simulink library "AEMS_Standard_Library"  (R2016b)
settings: Solver=ode45  StartTime=0.0  StopTime=10.0  RelTol=1e-3
undefined symbols (not defined in the file or in its folder): BkPY, carto, Cbx_extegr, Cbx_lpegrsys, Cbx_portegr, Cnx_bnk_nr_conf, Cnx_cyl_nr_conf, ConfigManagement, configuration_management, Cxx_dcm_io_tmr_end_xxxx, Cxx_dcm_rt_tmr_end, Cxx_DID_xxxx_IO_max, Cxx_DID_xxxx_IO_min, Cxx_egrhsofs, Cxx_vmaniegi, DEM_DEBOUNCE_FREEZE, DEM_DTR_CTL_INVISIBLE, DEM_DTR_CTL_NORMAL, Dem_DtrId2_XXX, Dem_DtrId3_XXX, Dem_DtrId4_XXX, Dem_DtrId5_XXX, Dem_DtrId6_XXX, Dem_DtrId7_XXX, Dem_DtrId8_XXX, Dem_DtrId9_XXX, Dem_DtrId_XXX, Dem_EnableConditionId2_XXX, Dem_EnableConditionId3_XXX, Dem_EnableConditionId4_XXX, Dem_EnableConditionId5_XXX, Dem_EnableConditionId6_XXX, Dem_EnableConditionId7_XXX, Dem_EnableConditionId8_XXX, Dem_EnableConditionId_XXX, Dem_EventId, Dem_EventId2_XXX, Dem_EventId3_XXX, Dem_EventId4_XXX, Dem_EventId5_XXX, Dem_EventId6_XXX, Dem_EventId7_XXX, Dem_EventId8_XXX, Dem_EventId9_XXX, Dem_EventId_Device_Faulttype, Dem_EventId_XXX, DEM_IUMPR_GENERAL_DENOMINATOR, DEM_OPCYC_IGNITION, Dem_RatioId2_XXX, Dem_RatioId3_XXX, Dem_RatioId4_XXX, Dem_RatioId5_XXX, Dem_RatioId6_XXX, Dem_RatioId7_XXX, Dem_RatioId8_XXX, Dem_RatioId_XXX, Dem_StorageConditionId2_XXX, Dem_StorageConditionId3_XXX, Dem_StorageConditionId4_XXX, Dem_StorageConditionId5_XXX ... (+65)
libraries: AEMS_Standard_Library x477, simulink x2
(part 29 of 39)

== system AEMS_Standard_Library/SUB/AEMS_DEM_COUNTER_BASED_DEBOUNCE_1D/AEMS_DEM_COUNTER_BASED_DEBOUNCE_CALL ==
  conditionfulfilled : Inport
  prefailed : Inport  Port=2
  prepassed : Inport  Port=3
  reseteventdebounce : Inport  Port=4
  DemDebounceBehavior : Inport  Port=5
  DemCounterFailedThreshold : Inport  Port=6
  DemCounterIncrementStepSize : Inport  Port=7
  DemCounterJumpUp : Inport  Port=8
  DemCounterJumpUpValue : Inport  Port=9
  DemCounterPassedThreshold : Inport  Port=10
  DemCounterDecrementStepSize : Inport  Port=11
  DemCounterJumpDown : Inport  Port=12
  DemCounterJumpDownValue : Inport  Port=13
  Enable : EnablePort
      settings: AttributesFormatString=StatesWhenEnabling = %<StatesWhenEnabling>
  AEMS_DEM_COUNTERBASEDDEBOUNCE : AEMS_Standard_Library/SUB/AEMS_DEM_COUNTERBASEDDEBOUNCE  Tag=[LIB]  eventid=Dem_EventId_Device_Faulttype
      settings: AttributesFormatString=|
      | %<MaskType>
      | EventId: %<eventid>
  debouncevalue : Outport
      settings: AttributesFormatString=<initial=%<InitialOutput>>\n<whendisabled=%<OutputWhenDisabled>>
  failed : Outport  Port=2
      settings: AttributesFormatString=<initial=%<InitialOutput>>\n<whendisabled=%<OutputWhenDisabled>>
  passed : Outport  Port=3
      settings: AttributesFormatString=<initial=%<InitialOutput>>\n<whendisabled=%<OutputWhenDisabled>>
  wires:
  DemCounterJumpDownValue/1 -> AEMS_DEM_COUNTERBASEDDEBOUNCE/13
  DemCounterJumpDown/1 -> AEMS_DEM_COUNTERBASEDDEBOUNCE/12
  DemCounterDecrementStepSize/1 -> AEMS_DEM_COUNTERBASEDDEBOUNCE/11
  DemCounterPassedThreshold/1 -> AEMS_DEM_COUNTERBASEDDEBOUNCE/10
  DemCounterJumpUpValue/1 -> AEMS_DEM_COUNTERBASEDDEBOUNCE/9
  DemCounterJumpUp/1 -> AEMS_DEM_COUNTERBASEDDEBOUNCE/8
  DemCounterIncrementStepSize/1 -> AEMS_DEM_COUNTERBASEDDEBOUNCE/7
  DemCounterFailedThreshold/1 -> AEMS_DEM_COUNTERBASEDDEBOUNCE/6
  DemDebounceBehavior/1 -> AEMS_DEM_COUNTERBASEDDEBOUNCE/5
  reseteventdebounce/1 -> AEMS_DEM_COUNTERBASEDDEBOUNCE/4
  AEMS_DEM_COUNTERBASEDDEBOUNCE/3 -> passed/1
  AEMS_DEM_COUNTERBASEDDEBOUNCE/2 -> failed/1
  AEMS_DEM_COUNTERBASEDDEBOUNCE/1 -> debouncevalue/1
  prefailed/1 -> AEMS_DEM_COUNTERBASEDDEBOUNCE/2
  prepassed/1 -> AEMS_DEM_COUNTERBASEDDEBOUNCE/3
  conditionfulfilled/1 -> AEMS_DEM_COUNTERBASEDDEBOUNCE/1

== system AEMS_Standard_Library/SUB/AEMS_DEM_COUNTER_BASED_DEBOUNCE_2D/AEMS_DEM_COUNTER_BASED_DEBOUNCE_CALL1 ==
  conditionfulfilled : Inport
  prefailed : Inport  Port=2
  prepassed : Inport  Port=3
  reseteventdebounce : Inport  Port=4
  DemDebounceBehavior : Inport  Port=5
  DemCounterFailedThreshold : Inport  Port=6
  DemCounterIncrementStepSize : Inport  Port=7
  DemCounterJumpUp : Inport  Port=8
  DemCounterJumpUpValue : Inport  Port=9
  DemCounterPassedThreshold : Inport  Port=10
  DemCounterDecrementStepSize : Inport  Port=11
  DemCounterJumpDown : Inport  Port=12
  DemCounterJumpDownValue : Inport  Port=13
  Enable : EnablePort
  AEMS_DEM_COUNTERBASEDDEBOUNCE : AEMS_Standard_Library/SUB/AEMS_DEM_COUNTERBASEDDEBOUNCE  Tag=[LIB]  eventid=Dem_EventId_Device_Faulttype
      settings: AttributesFormatString=|
      | %<MaskType>
      | EventId: %<eventid>
  debouncevalue : Outport
  failed : Outport  Port=2
  passed : Outport  Port=3
  wires:
  DemCounterJumpDown/1 -> AEMS_DEM_COUNTERBASEDDEBOUNCE/12
  DemCounterJumpDownValue/1 -> AEMS_DEM_COUNTERBASEDDEBOUNCE/13
  DemDebounceBehavior/1 -> AEMS_DEM_COUNTERBASEDDEBOUNCE/5
  DemCounterFailedThreshold/1 -> AEMS_DEM_COUNTERBASEDDEBOUNCE/6
  DemCounterJumpUpValue/1 -> AEMS_DEM_COUNTERBASEDDEBOUNCE/9
  DemCounterIncrementStepSize/1 -> AEMS_DEM_COUNTERBASEDDEBOUNCE/7
  DemCounterJumpUp/1 -> AEMS_DEM_COUNTERBASEDDEBOUNCE/8
  DemCounterPassedThreshold/1 -> AEMS_DEM_COUNTERBASEDDEBOUNCE/10
  DemCounterDecrementStepSize/1 -> AEMS_DEM_COUNTERBASEDDEBOUNCE/11
  reseteventdebounce/1 -> AEMS_DEM_COUNTERBASEDDEBOUNCE/4
  conditionfulfilled/1 -> AEMS_DEM_COUNTERBASEDDEBOUNCE/1
  prepassed/1 -> AEMS_DEM_COUNTERBASEDDEBOUNCE/3
  prefailed/1 -> AEMS_DEM_COUNTERBASEDDEBOUNCE/2
  AEMS_DEM_COUNTERBASEDDEBOUNCE/1 -> debouncevalue/1
  AEMS_DEM_COUNTERBASEDDEBOUNCE/2 -> failed/1
  AEMS_DEM_COUNTERBASEDDEBOUNCE/3 -> passed/1

== system AEMS_Standard_Library/SUB/AEMS_DEM_COUNTER_BASED_DEBOUNCE_2D/AEMS_DEM_COUNTER_BASED_DEBOUNCE_CALL2 ==
  conditionfulfilled : Inport
  prefailed : Inport  Port=2
  prepassed : Inport  Port=3
  reseteventdebounce : Inport  Port=4
  DemDebounceBehavior : Inport  Port=5
  DemCounterFailedThreshold : Inport  Port=6
  DemCounterIncrementStepSize : Inport  Port=7
  DemCounterJumpUp : Inport  Port=8
  DemCounterJumpUpValue : Inport  Port=9
  DemCounterPassedThreshold : Inport  Port=10
  DemCounterDecrementStepSize : Inport  Port=11
  DemCounterJumpDown : Inport  Port=12
  DemCounterJumpDownValue : Inport  Port=13
  Enable : EnablePort
  AEMS_DEM_COUNTERBASEDDEBOUNCE : AEMS_Standard_Library/SUB/AEMS_DEM_COUNTERBASEDDEBOUNCE  Tag=[LIB]  eventid=Dem_EventId_Device2_Faulttype
      settings: AttributesFormatString=|
      | %<MaskType>
      | EventId: %<eventid>
  debouncevalue : Outport
  failed : Outport  Port=2
  passed : Outport  Port=3
  wires:
  DemCounterJumpDownValue/1 -> AEMS_DEM_COUNTERBASEDDEBOUNCE/13
  DemCounterJumpDown/1 -> AEMS_DEM_COUNTERBASEDDEBOUNCE/12
  DemCounterDecrementStepSize/1 -> AEMS_DEM_COUNTERBASEDDEBOUNCE/11
  DemCounterPassedThreshold/1 -> AEMS_DEM_COUNTERBASEDDEBOUNCE/10
  DemCounterJumpUpValue/1 -> AEMS_DEM_COUNTERBASEDDEBOUNCE/9
  DemCounterJumpUp/1 -> AEMS_DEM_COUNTERBASEDDEBOUNCE/8
  DemCounterIncrementStepSize/1 -> AEMS_DEM_COUNTERBASEDDEBOUNCE/7
  DemCounterFailedThreshold/1 -> AEMS_DEM_COUNTERBASEDDEBOUNCE/6
  DemDebounceBehavior/1 -> AEMS_DEM_COUNTERBASEDDEBOUNCE/5
  reseteventdebounce/1 -> AEMS_DEM_COUNTERBASEDDEBOUNCE/4
  conditionfulfilled/1 -> AEMS_DEM_COUNTERBASEDDEBOUNCE/1
  prepassed/1 -> AEMS_DEM_COUNTERBASEDDEBOUNCE/3
  prefailed/1 -> AEMS_DEM_COUNTERBASEDDEBOUNCE/2
  AEMS_DEM_COUNTERBASEDDEBOUNCE/1 -> debouncevalue/1
  AEMS_DEM_COUNTERBASEDDEBOUNCE/2 -> failed/1
  AEMS_DEM_COUNTERBASEDDEBOUNCE/3 -> passed/1

== system AEMS_Standard_Library/SUB/AEMS_DEM_COUNTER_BASED_DEBOUNCE_3D/AEMS_DEM_COUNTER_BASED_DEBOUNCE_CALL1 ==
  conditionfulfilled : Inport
  prefailed : Inport  Port=2
  prepassed : Inport  Port=3
  reseteventdebounce : Inport  Port=4
  DemDebounceBehavior : Inport  Port=5
  DemCounterFailedThreshold : Inport  Port=6
  DemCounterIncrementStepSize : Inport  Port=7
  DemCounterJumpUp : Inport  Port=8
  DemCounterJumpUpValue : Inport  Port=9
  DemCounterPassedThreshold : Inport  Port=10
  DemCounterDecrementStepSize : Inport  Port=11
  DemCounterJumpDown : Inport  Port=12
  DemCounterJumpDownValue : Inport  Port=13
  Enable : EnablePort
  AEMS_DEM_COUNTERBASEDDEBOUNCE : AEMS_Standard_Library/SUB/AEMS_DEM_COUNTERBASEDDEBOUNCE  Tag=[LIB]  eventid=Dem_EventId_Device_Faulttype
      settings: AttributesFormatString=|
      | %<MaskType>
      | EventId: %<eventid>
  debouncevalue : Outport
  failed : Outport  Port=2
  passed : Outport  Port=3
  wires:
  DemDebounceBehavior/1 -> AEMS_DEM_COUNTERBASEDDEBOUNCE/5
  DemCounterIncrementStepSize/1 -> AEMS_DEM_COUNTERBASEDDEBOUNCE/7
  DemCounterFailedThreshold/1 -> AEMS_DEM_COUNTERBASEDDEBOUNCE/6
  DemCounterJumpUp/1 -> AEMS_DEM_COUNTERBASEDDEBOUNCE/8
  DemCounterPassedThreshold/1 -> AEMS_DEM_COUNTERBASEDDEBOUNCE/10
  DemCounterJumpUpValue/1 -> AEMS_DEM_COUNTERBASEDDEBOUNCE/9
  DemCounterDecrementStepSize/1 -> AEMS_DEM_COUNTERBASEDDEBOUNCE/11
  DemCounterJumpDownValue/1 -> AEMS_DEM_COUNTERBASEDDEBOUNCE/13
  DemCounterJumpDown/1 -> AEMS_DEM_COUNTERBASEDDEBOUNCE/12
  reseteventdebounce/1 -> AEMS_DEM_COUNTERBASEDDEBOUNCE/4
  conditionfulfilled/1 -> AEMS_DEM_COUNTERBASEDDEBOUNCE/1
  prepassed/1 -> AEMS_DEM_COUNTERBASEDDEBOUNCE/3
  prefailed/1 -> AEMS_DEM_COUNTERBASEDDEBOUNCE/2
  AEMS_DEM_COUNTERBASEDDEBOUNCE/1 -> debouncevalue/1
  AEMS_DEM_COUNTERBASEDDEBOUNCE/2 -> failed/1
  AEMS_DEM_COUNTERBASEDDEBOUNCE/3 -> passed/1

== system AEMS_Standard_Library/SUB/AEMS_DEM_COUNTER_BASED_DEBOUNCE_3D/AEMS_DEM_COUNTER_BASED_DEBOUNCE_CALL2 ==
  conditionfulfilled : Inport
  prefailed : Inport  Port=2
  prepassed : Inport  Port=3
  reseteventdebounce : Inport  Port=4
  DemDebounceBehavior : Inport  Port=5
  DemCounterFailedThreshold : Inport  Port=6
  DemCounterIncrementStepSize : Inport  Port=7
  DemCounterJumpUp : Inport  Port=8
  DemCounterJumpUpValue : Inport  Port=9
  DemCounterPassedThreshold : Inport  Port=10
  DemCounterDecrementStepSize : Inport  Port=11
  DemCounterJumpDown : Inport  Port=12
  DemCounterJumpDownValue : Inport  Port=13
  Enable : EnablePort
  AEMS_DEM_COUNTERBASEDDEBOUNCE : AEMS_Standard_Library/SUB/AEMS_DEM_COUNTERBASEDDEBOUNCE  Tag=[LIB]  eventid=Dem_EventId_Device2_Faulttype
      settings: AttributesFormatString=|
      | %<MaskType>
      | EventId: %<eventid>
  debouncevalue : Outport
  failed : Outport  Port=2
  passed : Outport  Port=3
  wires:
  DemDebounceBehavior/1 -> AEMS_DEM_COUNTERBASEDDEBOUNCE/5
  DemCounterIncrementStepSize/1 -> AEMS_DEM_COUNTERBASEDDEBOUNCE/7
  DemCounterFailedThreshold/1 -> AEMS_DEM_COUNTERBASEDDEBOUNCE/6
  DemCounterJumpUp/1 -> AEMS_DEM_COUNTERBASEDDEBOUNCE/8
  DemCounterPassedThreshold/1 -> AEMS_DEM_COUNTERBASEDDEBOUNCE/10
  DemCounterJumpUpValue/1 -> AEMS_DEM_COUNTERBASEDDEBOUNCE/9
  DemCounterDecrementStepSize/1 -> AEMS_DEM_COUNTERBASEDDEBOUNCE/11
  DemCounterJumpDownValue/1 -> AEMS_DEM_COUNTERBASEDDEBOUNCE/13
  DemCounterJumpDown/1 -> AEMS_DEM_COUNTERBASEDDEBOUNCE/12
  reseteventdebounce/1 -> AEMS_DEM_COUNTERBASEDDEBOUNCE/4
  conditionfulfilled/1 -> AEMS_DEM_COUNTERBASEDDEBOUNCE/1
  prepassed/1 -> AEMS_DEM_COUNTERBASEDDEBOUNCE/3
  prefailed/1 -> AEMS_DEM_COUNTERBASEDDEBOUNCE/2
  AEMS_DEM_COUNTERBASEDDEBOUNCE/1 -> debouncevalue/1
  AEMS_DEM_COUNTERBASEDDEBOUNCE/2 -> failed/1
  AEMS_DEM_COUNTERBASEDDEBOUNCE/3 -> passed/1

== system AEMS_Standard_Library/SUB/AEMS_DEM_COUNTER_BASED_DEBOUNCE_3D/AEMS_DEM_COUNTER_BASED_DEBOUNCE_CALL3 ==
  conditionfulfilled : Inport
  prefailed : Inport  Port=2
  prepassed : Inport  Port=3
  reseteventdebounce : Inport  Port=4
  DemDebounceBehavior : Inport  Port=5
  DemCounterFailedThreshold : Inport  Port=6
  DemCounterIncrementStepSize : Inport  Port=7
  DemCounterJumpUp : Inport  Port=8
  DemCounterJumpUpValue : Inport  Port=9
  DemCounterPassedThreshold : Inport  Port=10
  DemCounterDecrementStepSize : Inport  Port=11
  DemCounterJumpDown : Inport  Port=12
  DemCounterJumpDownValue : Inport  Port=13
  Enable : EnablePort
  AEMS_DEM_COUNTERBASEDDEBOUNCE : AEMS_Standard_Library/SUB/AEMS_DEM_COUNTERBASEDDEBOUNCE  Tag=[LIB]  eventid=Dem_EventId_Device3_Faulttype
      settings: AttributesFormatString=|
      | %<MaskType>
      | EventId: %<eventid>
  debouncevalue : Outport
  failed : Outport  Port=2
  passed : Outport  Port=3
  wires:
  DemCounterJumpDownValue/1 -> AEMS_DEM_COUNTERBASEDDEBOUNCE/13
  DemDebounceBehavior/1 -> AEMS_DEM_COUNTERBASEDDEBOUNCE/5
  DemCounterFailedThreshold/1 -> AEMS_DEM_COUNTERBASEDDEBOUNCE/6
  DemCounterIncrementStepSize/1 -> AEMS_DEM_COUNTERBASEDDEBOUNCE/7
  DemCounterJumpUp/1 -> AEMS_DEM_COUNTERBASEDDEBOUNCE/8
  DemCounterJumpUpValue/1 -> AEMS_DEM_COUNTERBASEDDEBOUNCE/9
  DemCounterPassedThreshold/1 -> AEMS_DEM_COUNTERBASEDDEBOUNCE/10
  DemCounterDecrementStepSize/1 -> AEMS_DEM_COUNTERBASEDDEBOUNCE/11
  DemCounterJumpDown/1 -> AEMS_DEM_COUNTERBASEDDEBOUNCE/12
  reseteventdebounce/1 -> AEMS_DEM_COUNTERBASEDDEBOUNCE/4
  AEMS_DEM_COUNTERBASEDDEBOUNCE/3 -> passed/1
  AEMS_DEM_COUNTERBASEDDEBOUNCE/2 -> failed/1
  AEMS_DEM_COUNTERBASEDDEBOUNCE/1 -> debouncevalue/1
  prefailed/1 -> AEMS_DEM_COUNTERBASEDDEBOUNCE/2
  prepassed/1 -> AEMS_DEM_COUNTERBASEDDEBOUNCE/3
  conditionfulfilled/1 -> AEMS_DEM_COUNTERBASEDDEBOUNCE/1

== system AEMS_Standard_Library/SUB/AEMS_DEM_COUNTER_BASED_DEBOUNCE_4D/AEMS_DEM_COUNTER_BASED_DEBOUNCE_CALL1 ==
  conditionfulfilled : Inport
  prefailed : Inport  Port=2
  prepassed : Inport  Port=3
  reseteventdebounce : Inport  Port=4
  DemDebounceBehavior : Inport  Port=5
  DemCounterFailedThreshold : Inport  Port=6
  DemCounterIncrementStepSize : Inport  Port=7
  DemCounterJumpUp : Inport  Port=8
  DemCounterJumpUpValue : Inport  Port=9
  DemCounterPassedThreshold : Inport  Port=10
  DemCounterDecrementStepSize : Inport  Port=11
  DemCounterJumpDown : Inport  Port=12
  DemCounterJumpDownValue : Inport  Port=13
  Enable : EnablePort
  AEMS_DEM_COUNTERBASEDDEBOUNCE : AEMS_Standard_Library/SUB/AEMS_DEM_COUNTERBASEDDEBOUNCE  Tag=[LIB]  eventid=Dem_EventId_Device_Faulttype
      settings: AttributesFormatString=|
      | %<MaskType>
      | EventId: %<eventid>
  debouncevalue : Outport
  failed : Outport  Port=2
  passed : Outport  Port=3
  wires:
  reseteventdebounce/1 -> AEMS_DEM_COUNTERBASEDDEBOUNCE/4
  DemCounterIncrementStepSize/1 -> AEMS_DEM_COUNTERBASEDDEBOUNCE/7
  DemCounterJumpUpValue/1 -> AEMS_DEM_COUNTERBASEDDEBOUNCE/9
  DemDebounceBehavior/1 -> AEMS_DEM_COUNTERBASEDDEBOUNCE/5
  DemCounterJumpUp/1 -> AEMS_DEM_COUNTERBASEDDEBOUNCE/8
  DemCounterDecrementStepSize/1 -> AEMS_DEM_COUNTERBASEDDEBOUNCE/11
  DemCounterPassedThreshold/1 -> AEMS_DEM_COUNTERBASEDDEBOUNCE/10
  DemCounterFailedThreshold/1 -> AEMS_DEM_COUNTERBASEDDEBOUNCE/6
  DemCounterJumpDown/1 -> AEMS_DEM_COUNTERBASEDDEBOUNCE/12
  DemCounterJumpDownValue/1 -> AEMS_DEM_COUNTERBASEDDEBOUNCE/13
  AEMS_DEM_COUNTERBASEDDEBOUNCE/3 -> passed/1
  AEMS_DEM_COUNTERBASEDDEBOUNCE/2 -> failed/1
  AEMS_DEM_COUNTERBASEDDEBOUNCE/1 -> debouncevalue/1
  prefailed/1 -> AEMS_DEM_COUNTERBASEDDEBOUNCE/2
  prepassed/1 -> AEMS_DEM_COUNTERBASEDDEBOUNCE/3
  conditionfulfilled/1 -> AEMS_DEM_COUNTERBASEDDEBOUNCE/1

== system AEMS_Standard_Library/SUB/AEMS_DEM_COUNTER_BASED_DEBOUNCE_4D/AEMS_DEM_COUNTER_BASED_DEBOUNCE_CALL2 ==
  conditionfulfilled : Inport
  prefailed : Inport  Port=2
  prepassed : Inport  Port=3
  reseteventdebounce : Inport  Port=4
  DemDebounceBehavior : Inport  Port=5
  DemCounterFailedThreshold : Inport  Port=6
  DemCounterIncrementStepSize : Inport  Port=7
  DemCounterJumpUp : Inport  Port=8
  DemCounterJumpUpValue : Inport  Port=9
  DemCounterPassedThreshold : Inport  Port=10
  DemCounterDecrementStepSize : Inport  Port=11
  DemCounterJumpDown : Inport  Port=12
  DemCounterJumpDownValue : Inport  Port=13
  Enable : EnablePort
  AEMS_DEM_COUNTERBASEDDEBOUNCE : AEMS_Standard_Library/SUB/AEMS_DEM_COUNTERBASEDDEBOUNCE  Tag=[LIB]  eventid=Dem_EventId_Device2_Faulttype
      settings: AttributesFormatString=|
      | %<MaskType>
      | EventId: %<eventid>
  debouncevalue : Outport
  failed : Outport  Port=2
  passed : Outport  Port=3
  wires:
  DemCounterIncrementStepSize/1 -> AEMS_DEM_COUNTERBASEDDEBOUNCE/7
  DemDebounceBehavior/1 -> AEMS_DEM_COUNTERBASEDDEBOUNCE/5
  DemCounterJumpUpValue/1 -> AEMS_DEM_COUNTERBASEDDEBOUNCE/9
  DemCounterFailedThreshold/1 -> AEMS_DEM_COUNTERBASEDDEBOUNCE/6
  DemCounterJumpUp/1 -> AEMS_DEM_COUNTERBASEDDEBOUNCE/8
  DemCounterDecrementStepSize/1 -> AEMS_DEM_COUNTERBASEDDEBOUNCE/11
  DemCounterPassedThreshold/1 -> AEMS_DEM_COUNTERBASEDDEBOUNCE/10
  DemCounterJumpDownValue/1 -> AEMS_DEM_COUNTERBASEDDEBOUNCE/13
  DemCounterJumpDown/1 -> AEMS_DEM_COUNTERBASEDDEBOUNCE/12
  reseteventdebounce/1 -> AEMS_DEM_COUNTERBASEDDEBOUNCE/4
  AEMS_DEM_COUNTERBASEDDEBOUNCE/3 -> passed/1
  AEMS_DEM_COUNTERBASEDDEBOUNCE/2 -> failed/1
  AEMS_DEM_COUNTERBASEDDEBOUNCE/1 -> debouncevalue/1
  prefailed/1 -> AEMS_DEM_COUNTERBASEDDEBOUNCE/2
  prepassed/1 -> AEMS_DEM_COUNTERBASEDDEBOUNCE/3
  conditionfulfilled/1 -> AEMS_DEM_COUNTERBASEDDEBOUNCE/1

== system AEMS_Standard_Library/SUB/AEMS_DEM_COUNTER_BASED_DEBOUNCE_4D/AEMS_DEM_COUNTER_BASED_DEBOUNCE_CALL3 ==
  conditionfulfilled : Inport
  prefailed : Inport  Port=2
  prepassed : Inport  Port=3
  reseteventdebounce : Inport  Port=4
  DemDebounceBehavior : Inport  Port=5
  DemCounterFailedThreshold : Inport  Port=6
  DemCounterIncrementStepSize : Inport  Port=7
  DemCounterJumpUp : Inport  Port=8
  DemCounterJumpUpValue : Inport  Port=9
  DemCounterPassedThreshold : Inport  Port=10
  DemCounterDecrementStepSize : Inport  Port=11
  DemCounterJumpDown : Inport  Port=12
  DemCounterJumpDownValue : Inport  Port=13
  Enable : EnablePort
  AEMS_DEM_COUNTERBASEDDEBOUNCE : AEMS_Standard_Library/SUB/AEMS_DEM_COUNTERBASEDDEBOUNCE  Tag=[LIB]  eventid=Dem_EventId_Device3_Faulttype
      settings: AttributesFormatString=|
      | %<MaskType>
      | EventId: %<eventid>
  debouncevalue : Outport
  failed : Outport  Port=2
  passed : Outport  Port=3
  wires:
  reseteventdebounce/1 -> AEMS_DEM_COUNTERBASEDDEBOUNCE/4
  DemCounterJumpDown/1 -> AEMS_DEM_COUNTERBASEDDEBOUNCE/12
  DemCounterPassedThreshold/1 -> AEMS_DEM_COUNTERBASEDDEBOUNCE/10
  DemDebounceBehavior/1 -> AEMS_DEM_COUNTERBASEDDEBOUNCE/5
  DemCounterJumpUpValue/1 -> AEMS_DEM_COUNTERBASEDDEBOUNCE/9
  DemCounterDecrementStepSize/1 -> AEMS_DEM_COUNTERBASEDDEBOUNCE/11
  DemCounterFailedThreshold/1 -> AEMS_DEM_COUNTERBASEDDEBOUNCE/6
  DemCounterIncrementStepSize/1 -> AEMS_DEM_COUNTERBASEDDEBOUNCE/7
  DemCounterJumpDownValue/1 -> AEMS_DEM_COUNTERBASEDDEBOUNCE/13
  DemCounterJumpUp/1 -> AEMS_DEM_COUNTERBASEDDEBOUNCE/8
  conditionfulfilled/1 -> AEMS_DEM_COUNTERBASEDDEBOUNCE/1
  prepassed/1 -> AEMS_DEM_COUNTERBASEDDEBOUNCE/3
  prefailed/1 -> AEMS_DEM_COUNTERBASEDDEBOUNCE/2
  AEMS_DEM_COUNTERBASEDDEBOUNCE/1 -> debouncevalue/1
  AEMS_DEM_COUNTERBASEDDEBOUNCE/2 -> failed/1
  AEMS_DEM_COUNTERBASEDDEBOUNCE/3 -> passed/1

== system AEMS_Standard_Library/SUB/AEMS_DEM_COUNTER_BASED_DEBOUNCE_4D/AEMS_DEM_COUNTER_BASED_DEBOUNCE_CALL4 ==
  conditionfulfilled : Inport
  prefailed : Inport  Port=2
  prepassed : Inport  Port=3
  reseteventdebounce : Inport  Port=4
  DemDebounceBehavior : Inport  Port=5
  DemCounterFailedThreshold : Inport  Port=6
  DemCounterIncrementStepSize : Inport  Port=7
  DemCounterJumpUp : Inport  Port=8
  DemCounterJumpUpValue : Inport  Port=9
  DemCounterPassedThreshold : Inport  Port=10
  DemCounterDecrementStepSize : Inport  Port=11
  DemCounterJumpDown : Inport  Port=12
  DemCounterJumpDownValue : Inport  Port=13
  Enable : EnablePort
  AEMS_DEM_COUNTERBASEDDEBOUNCE : AEMS_Standard_Library/SUB/AEMS_DEM_COUNTERBASEDDEBOUNCE  Tag=[LIB]  eventid=Dem_EventId_Device4_Faulttype
      settings: AttributesFormatString=|
      | %<MaskType>
      | EventId: %<eventid>
  debouncevalue : Outport
  failed : Outport  Port=2
  passed : Outport  Port=3
  wires:
  DemCounterDecrementStepSize/1 -> AEMS_DEM_COUNTERBASEDDEBOUNCE/11
  DemCounterJumpDown/1 -> AEMS_DEM_COUNTERBASEDDEBOUNCE/12
  DemDebounceBehavior/1 -> AEMS_DEM_COUNTERBASEDDEBOUNCE/5
  DemCounterFailedThreshold/1 -> AEMS_DEM_COUNTERBASEDDEBOUNCE/6
  reseteventdebounce/1 -> AEMS_DEM_COUNTERBASEDDEBOUNCE/4
  DemCounterIncrementStepSize/1 -> AEMS_DEM_COUNTERBASEDDEBOUNCE/7
  DemCounterJumpUpValue/1 -> AEMS_DEM_COUNTERBASEDDEBOUNCE/9
  DemCounterJumpDownValue/1 -> AEMS_DEM_COUNTERBASEDDEBOUNCE/13
  DemCounterJumpUp/1 -> AEMS_DEM_COUNTERBASEDDEBOUNCE/8
  DemCounterPassedThreshold/1 -> AEMS_DEM_COUNTERBASEDDEBOUNCE/10
  AEMS_DEM_COUNTERBASEDDEBOUNCE/3 -> passed/1
  AEMS_DEM_COUNTERBASEDDEBOUNCE/2 -> failed/1
  AEMS_DEM_COUNTERBASEDDEBOUNCE/1 -> debouncevalue/1
  prefailed/1 -> AEMS_DEM_COUNTERBASEDDEBOUNCE/2
  prepassed/1 -> AEMS_DEM_COUNTERBASEDDEBOUNCE/3
  conditionfulfilled/1 -> AEMS_DEM_COUNTERBASEDDEBOUNCE/1

== system AEMS_Standard_Library/SUB/AEMS_DEM_COUNTER_BASED_DEBOUNCE_6D/AEMS_DEM_COUNTER_BASED_DEBOUNCE_CALL1 ==
  conditionfulfilled : Inport
  prefailed : Inport  Port=2
  prepassed : Inport  Port=3
  reseteventdebounce : Inport  Port=4
  DemDebounceBehavior : Inport  Port=5
  DemCounterFailedThreshold : Inport  Port=6
  DemCounterIncrementStepSize : Inport  Port=7
  DemCounterJumpUp : Inport  Port=8
  DemCounterJumpUpValue : Inport  Port=9
  DemCounterPassedThreshold : Inport  Port=10
  DemCounterDecrementStepSize : Inport  Port=11
  DemCounterJumpDown : Inport  Port=12
  DemCounterJumpDownValue : Inport  Port=13
  Enable : EnablePort
  AEMS_DEM_COUNTERBASEDDEBOUNCE : AEMS_Standard_Library/SUB/AEMS_DEM_COUNTERBASEDDEBOUNCE  Tag=[LIB]  eventid=Dem_EventId_Device_Faulttype
      settings: AttributesFormatString=|
      | %<MaskType>
      | EventId: %<eventid>
  debouncevalue : Outport
  failed : Outport  Port=2
  passed : Outport  Port=3
  wires:
  DemCounterJumpUp/1 -> AEMS_DEM_COUNTERBASEDDEBOUNCE/8
  DemCounterIncrementStepSize/1 -> AEMS_DEM_COUNTERBASEDDEBOUNCE/7
  DemCounterJumpUpValue/1 -> AEMS_DEM_COUNTERBASEDDEBOUNCE/9
  DemCounterFailedThreshold/1 -> AEMS_DEM_COUNTERBASEDDEBOUNCE/6
  DemDebounceBehavior/1 -> AEMS_DEM_COUNTERBASEDDEBOUNCE/5
  DemCounterJumpDownValue/1 -> AEMS_DEM_COUNTERBASEDDEBOUNCE/13
  DemCounterJumpDown/1 -> AEMS_DEM_COUNTERBASEDDEBOUNCE/12
  DemCounterDecrementStepSize/1 -> AEMS_DEM_COUNTERBASEDDEBOUNCE/11
  DemCounterPassedThreshold/1 -> AEMS_DEM_COUNTERBASEDDEBOUNCE/10
  reseteventdebounce/1 -> AEMS_DEM_COUNTERBASEDDEBOUNCE/4
  AEMS_DEM_COUNTERBASEDDEBOUNCE/3 -> passed/1
  AEMS_DEM_COUNTERBASEDDEBOUNCE/2 -> failed/1
  AEMS_DEM_COUNTERBASEDDEBOUNCE/1 -> debouncevalue/1
  prefailed/1 -> AEMS_DEM_COUNTERBASEDDEBOUNCE/2
  prepassed/1 -> AEMS_DEM_COUNTERBASEDDEBOUNCE/3
  conditionfulfilled/1 -> AEMS_DEM_COUNTERBASEDDEBOUNCE/1

== system AEMS_Standard_Library/SUB/AEMS_DEM_COUNTER_BASED_DEBOUNCE_6D/AEMS_DEM_COUNTER_BASED_DEBOUNCE_CALL2 ==
  conditionfulfilled : Inport
  prefailed : Inport  Port=2
  prepassed : Inport  Port=3
  reseteventdebounce : Inport  Port=4
  DemDebounceBehavior : Inport  Port=5
  DemCounterFailedThreshold : Inport  Port=6
  DemCounterIncrementStepSize : Inport  Port=7
  DemCounterJumpUp : Inport  Port=8
  DemCounterJumpUpValue : Inport  Port=9
  DemCounterPassedThreshold : Inport  Port=10
  DemCounterDecrementStepSize : Inport  Port=11
  DemCounterJumpDown : Inport  Port=12
  DemCounterJumpDownValue : Inport  Port=13
  Enable : EnablePort
  AEMS_DEM_COUNTERBASEDDEBOUNCE : AEMS_Standard_Library/SUB/AEMS_DEM_COUNTERBASEDDEBOUNCE  Tag=[LIB]  eventid=Dem_EventId_Device2_Faulttype
      settings: AttributesFormatString=|
      | %<MaskType>
      | EventId: %<eventid>
  debouncevalue : Outport
  failed : Outport  Port=2
  passed : Outport  Port=3
  wires:
  reseteventdebounce/1 -> AEMS_DEM_COUNTERBASEDDEBOUNCE/4
  DemCounterJumpDownValue/1 -> AEMS_DEM_COUNTERBASEDDEBOUNCE/13
  DemCounterJumpDown/1 -> AEMS_DEM_COUNTERBASEDDEBOUNCE/12
  DemCounterDecrementStepSize/1 -> AEMS_DEM_COUNTERBASEDDEBOUNCE/11
  DemCounterPassedThreshold/1 -> AEMS_DEM_COUNTERBASEDDEBOUNCE/10
  DemCounterJumpUpValue/1 -> AEMS_DEM_COUNTERBASEDDEBOUNCE/9
  DemCounterJumpUp/1 -> AEMS_DEM_COUNTERBASEDDEBOUNCE/8
  DemCounterIncrementStepSize/1 -> AEMS_DEM_COUNTERBASEDDEBOUNCE/7
  DemCounterFailedThreshold/1 -> AEMS_DEM_COUNTERBASEDDEBOUNCE/6
  DemDebounceBehavior/1 -> AEMS_DEM_COUNTERBASEDDEBOUNCE/5
  AEMS_DEM_COUNTERBASEDDEBOUNCE/3 -> passed/1
  AEMS_DEM_COUNTERBASEDDEBOUNCE/2 -> failed/1
  AEMS_DEM_COUNTERBASEDDEBOUNCE/1 -> debouncevalue/1
  prefailed/1 -> AEMS_DEM_COUNTERBASEDDEBOUNCE/2
  prepassed/1 -> AEMS_DEM_COUNTERBASEDDEBOUNCE/3
  conditionfulfilled/1 -> AEMS_DEM_COUNTERBASEDDEBOUNCE/1

== system AEMS_Standard_Library/SUB/AEMS_DEM_COUNTER_BASED_DEBOUNCE_6D/AEMS_DEM_COUNTER_BASED_DEBOUNCE_CALL3 ==
  conditionfulfilled : Inport
  prefailed : Inport  Port=2
  prepassed : Inport  Port=3
  reseteventdebounce : Inport  Port=4
  DemDebounceBehavior : Inport  Port=5
  DemCounterFailedThreshold : Inport  Port=6
  DemCounterIncrementStepSize : Inport  Port=7
  DemCounterJumpUp : Inport  Port=8
  DemCounterJumpUpValue : Inport  Port=9
  DemCounterPassedThreshold : Inport  Port=10
  DemCounterDecrementStepSize : Inport  Port=11
  DemCounterJumpDown : Inport  Port=12
  DemCounterJumpDownValue : Inport  Port=13
  Enable : EnablePort
  AEMS_DEM_COUNTERBASEDDEBOUNCE : AEMS_Standard_Library/SUB/AEMS_DEM_COUNTERBASEDDEBOUNCE  Tag=[LIB]  eventid=Dem_EventId_Device3_Faulttype
      settings: AttributesFormatString=|
      | %<MaskType>
      | EventId: %<eventid>
  debouncevalue : Outport
  failed : Outport  Port=2
  passed : Outport  Port=3
  wires:
  DemCounterJumpDownValue/1 -> AEMS_DEM_COUNTERBASEDDEBOUNCE/13
  DemCounterJumpDown/1 -> AEMS_DEM_COUNTERBASEDDEBOUNCE/12
  DemCounterDecrementStepSize/1 -> AEMS_DEM_COUNTERBASEDDEBOUNCE/11
  DemCounterPassedThreshold/1 -> AEMS_DEM_COUNTERBASEDDEBOUNCE/10
  DemCounterJumpUpValue/1 -> AEMS_DEM_COUNTERBASEDDEBOUNCE/9
  DemCounterJumpUp/1 -> AEMS_DEM_COUNTERBASEDDEBOUNCE/8
  DemCounterIncrementStepSize/1 -> AEMS_DEM_COUNTERBASEDDEBOUNCE/7
  DemCounterFailedThreshold/1 -> AEMS_DEM_COUNTERBASEDDEBOUNCE/6
  DemDebounceBehavior/1 -> AEMS_DEM_COUNTERBASEDDEBOUNCE/5
  reseteventdebounce/1 -> AEMS_DEM_COUNTERBASEDDEBOUNCE/4
  conditionfulfilled/1 -> AEMS_DEM_COUNTERBASEDDEBOUNCE/1
  prepassed/1 -> AEMS_DEM_COUNTERBASEDDEBOUNCE/3
  prefailed/1 -> AEMS_DEM_COUNTERBASEDDEBOUNCE/2
  AEMS_DEM_COUNTERBASEDDEBOUNCE/1 -> debouncevalue/1
  AEMS_DEM_COUNTERBASEDDEBOUNCE/2 -> failed/1
  AEMS_DEM_COUNTERBASEDDEBOUNCE/3 -> passed/1

== system AEMS_Standard_Library/SUB/AEMS_DEM_COUNTER_BASED_DEBOUNCE_6D/AEMS_DEM_COUNTER_BASED_DEBOUNCE_CALL4 ==
  conditionfulfilled : Inport
  prefailed : Inport  Port=2
  prepassed : Inport  Port=3
  reseteventdebounce : Inport  Port=4
  DemDebounceBehavior : Inport  Port=5
  DemCounterFailedThreshold : Inport  Port=6
  DemCounterIncrementStepSize : Inport  Port=7
  DemCounterJumpUp : Inport  Port=8
  DemCounterJumpUpValue : Inport  Port=9
  DemCounterPassedThreshold : Inport  Port=10
  DemCounterDecrementStepSize : Inport  Port=11
  DemCounterJumpDown : Inport  Port=12
  DemCounterJumpDownValue : Inport  Port=13
  Enable : EnablePort
  AEMS_DEM_COUNTERBASEDDEBOUNCE : AEMS_Standard_Library/SUB/AEMS_DEM_COUNTERBASEDDEBOUNCE  Tag=[LIB]  eventid=Dem_EventId_Device4_Faulttype
      settings: AttributesFormatString=|
      | %<MaskType>
      | EventId: %<eventid>
  debouncevalue : Outport
  failed : Outport  Port=2
  passed : Outport  Port=3
  wires:
  DemCounterJumpDownValue/1 -> AEMS_DEM_COUNTERBASEDDEBOUNCE/13
  DemCounterJumpDown/1 -> AEMS_DEM_COUNTERBASEDDEBOUNCE/12
  DemCounterDecrementStepSize/1 -> AEMS_DEM_COUNTERBASEDDEBOUNCE/11
  DemCounterPassedThreshold/1 -> AEMS_DEM_COUNTERBASEDDEBOUNCE/10
  DemCounterJumpUpValue/1 -> AEMS_DEM_COUNTERBASEDDEBOUNCE/9
  DemCounterJumpUp/1 -> AEMS_DEM_COUNTERBASEDDEBOUNCE/8
  DemCounterIncrementStepSize/1 -> AEMS_DEM_COUNTERBASEDDEBOUNCE/7
  DemCounterFailedThreshold/1 -> AEMS_DEM_COUNTERBASEDDEBOUNCE/6
  DemDebounceBehavior/1 -> AEMS_DEM_COUNTERBASEDDEBOUNCE/5
  reseteventdebounce/1 -> AEMS_DEM_COUNTERBASEDDEBOUNCE/4
  AEMS_DEM_COUNTERBASEDDEBOUNCE/3 -> passed/1
  AEMS_DEM_COUNTERBASEDDEBOUNCE/2 -> failed/1
  AEMS_DEM_COUNTERBASEDDEBOUNCE/1 -> debouncevalue/1
  prefailed/1 -> AEMS_DEM_COUNTERBASEDDEBOUNCE/2
  prepassed/1 -> AEMS_DEM_COUNTERBASEDDEBOUNCE/3
  conditionfulfilled/1 -> AEMS_DEM_COUNTERBASEDDEBOUNCE/1

== system AEMS_Standard_Library/SUB/AEMS_DEM_COUNTER_BASED_DEBOUNCE_6D/AEMS_DEM_COUNTER_BASED_DEBOUNCE_CALL5 ==
  conditionfulfilled : Inport
  prefailed : Inport  Port=2
  prepassed : Inport  Port=3
  reseteventdebounce : Inport  Port=4
  DemDebounceBehavior : Inport  Port=5
  DemCounterFailedThreshold : Inport  Port=6
  DemCounterIncrementStepSize : Inport  Port=7
  DemCounterJumpUp : Inport  Port=8
  DemCounterJumpUpValue : Inport  Port=9
  DemCounterPassedThreshold : Inport  Port=10
  DemCounterDecrementStepSize : Inport  Port=11
  DemCounterJumpDown : Inport  Port=12
  DemCounterJumpDownValue : Inport  Port=13
  Enable : EnablePort
  AEMS_DEM_COUNTERBASEDDEBOUNCE : AEMS_Standard_Library/SUB/AEMS_DEM_COUNTERBASEDDEBOUNCE  Tag=[LIB]  eventid=Dem_EventId_Device5_Faulttype
      settings: AttributesFormatString=|
      | %<MaskType>
      | EventId: %<eventid>
  debouncevalue : Outport
  failed : Outport  Port=2
  passed : Outport  Port=3
  wires:
  DemCounterJumpDownValue/1 -> AEMS_DEM_COUNTERBASEDDEBOUNCE/13
  DemCounterJumpDown/1 -> AEMS_DEM_COUNTERBASEDDEBOUNCE/12
  DemCounterDecrementStepSize/1 -> AEMS_DEM_COUNTERBASEDDEBOUNCE/11
  DemCounterPassedThreshold/1 -> AEMS_DEM_COUNTERBASEDDEBOUNCE/10
  DemCounterJumpUpValue/1 -> AEMS_DEM_COUNTERBASEDDEBOUNCE/9
  DemCounterJumpUp/1 -> AEMS_DEM_COUNTERBASEDDEBOUNCE/8
  DemCounterIncrementStepSize/1 -> AEMS_DEM_COUNTERBASEDDEBOUNCE/7
  DemCounterFailedThreshold/1 -> AEMS_DEM_COUNTERBASEDDEBOUNCE/6
  DemDebounceBehavior/1 -> AEMS_DEM_COUNTERBASEDDEBOUNCE/5
  reseteventdebounce/1 -> AEMS_DEM_COUNTERBASEDDEBOUNCE/4
  AEMS_DEM_COUNTERBASEDDEBOUNCE/3 -> passed/1
  AEMS_DEM_COUNTERBASEDDEBOUNCE/2 -> failed/1
  AEMS_DEM_COUNTERBASEDDEBOUNCE/1 -> debouncevalue/1
  prefailed/1 -> AEMS_DEM_COUNTERBASEDDEBOUNCE/2
  prepassed/1 -> AEMS_DEM_COUNTERBASEDDEBOUNCE/3
  conditionfulfilled/1 -> AEMS_DEM_COUNTERBASEDDEBOUNCE/1

== system AEMS_Standard_Library/SUB/AEMS_DEM_COUNTER_BASED_DEBOUNCE_6D/AEMS_DEM_COUNTER_BASED_DEBOUNCE_CALL6 ==
  conditionfulfilled : Inport
  prefailed : Inport  Port=2
  prepassed : Inport  Port=3
  reseteventdebounce : Inport  Port=4
  DemDebounceBehavior : Inport  Port=5
  DemCounterFailedThreshold : Inport  Port=6
  DemCounterIncrementStepSize : Inport  Port=7
  DemCounterJumpUp : Inport  Port=8
  DemCounterJumpUpValue : Inport  Port=9
  DemCounterPassedThreshold : Inport  Port=10
  DemCounterDecrementStepSize : Inport  Port=11
  DemCounterJumpDown : Inport  Port=12
  DemCounterJumpDownValue : Inport  Port=13
  Enable : EnablePort
  AEMS_DEM_COUNTERBASEDDEBOUNCE : AEMS_Standard_Library/SUB/AEMS_DEM_COUNTERBASEDDEBOUNCE  Tag=[LIB]  eventid=Dem_EventId_Device6_Faulttype
      settings: AttributesFormatString=|
      | %<MaskType>
      | EventId: %<eventid>
  debouncevalue : Outport
  failed : Outport  Port=2
  passed : Outport  Port=3
  wires:
  DemCounterJumpDownValue/1 -> AEMS_DEM_COUNTERBASEDDEBOUNCE/13
  DemCounterJumpDown/1 -> AEMS_DEM_COUNTERBASEDDEBOUNCE/12
  DemCounterDecrementStepSize/1 -> AEMS_DEM_COUNTERBASEDDEBOUNCE/11
  DemCounterPassedThreshold/1 -> AEMS_DEM_COUNTERBASEDDEBOUNCE/10
  DemCounterJumpUpValue/1 -> AEMS_DEM_COUNTERBASEDDEBOUNCE/9
  DemCounterJumpUp/1 -> AEMS_DEM_COUNTERBASEDDEBOUNCE/8
  DemCounterIncrementStepSize/1 -> AEMS_DEM_COUNTERBASEDDEBOUNCE/7
  DemCounterFailedThreshold/1 -> AEMS_DEM_COUNTERBASEDDEBOUNCE/6
  DemDebounceBehavior/1 -> AEMS_DEM_COUNTERBASEDDEBOUNCE/5
  reseteventdebounce/1 -> AEMS_DEM_COUNTERBASEDDEBOUNCE/4
  AEMS_DEM_COUNTERBASEDDEBOUNCE/3 -> passed/1
  AEMS_DEM_COUNTERBASEDDEBOUNCE/2 -> failed/1
  AEMS_DEM_COUNTERBASEDDEBOUNCE/1 -> debouncevalue/1
  prefailed/1 -> AEMS_DEM_COUNTERBASEDDEBOUNCE/2
  prepassed/1 -> AEMS_DEM_COUNTERBASEDDEBOUNCE/3
  conditionfulfilled/1 -> AEMS_DEM_COUNTERBASEDDEBOUNCE/1

== system AEMS_Standard_Library/SUB/AEMS_DEM_COUNTER_BASED_DEBOUNCE_8D/AEMS_DEM_COUNTER_BASED_DEBOUNCE_CALL1 ==
  conditionfulfilled : Inport
  prefailed : Inport  Port=2
  prepassed : Inport  Port=3
  reseteventdebounce : Inport  Port=4
  DemDebounceBehavior : Inport  Port=5
  DemCounterFailedThreshold : Inport  Port=6
  DemCounterIncrementStepSize : Inport  Port=7
  DemCounterJumpUp : Inport  Port=8
  DemCounterJumpUpValue : Inport  Port=9
  DemCounterPassedThreshold : Inport  Port=10
  DemCounterDecrementStepSize : Inport  Port=11
  DemCounterJumpDown : Inport  Port=12
  DemCounterJumpDownValue : Inport  Port=13
  Enable : EnablePort
  AEMS_DEM_COUNTERBASEDDEBOUNCE : AEMS_Standard_Library/SUB/AEMS_DEM_COUNTERBASEDDEBOUNCE  Tag=[LIB]  eventid=Dem_EventId_Device_Faulttype
      settings: AttributesFormatString=|
      | %<MaskType>
      | EventId: %<eventid>
  debouncevalue : Outport
  failed : Outport  Port=2
  passed : Outport  Port=3
  wires:
  reseteventdebounce/1 -> AEMS_DEM_COUNTERBASEDDEBOUNCE/4
  DemDebounceBehavior/1 -> AEMS_DEM_COUNTERBASEDDEBOUNCE/5
  DemCounterFailedThreshold/1 -> AEMS_DEM_COUNTERBASEDDEBOUNCE/6
  DemCounterJumpDown/1 -> AEMS_DEM_COUNTERBASEDDEBOUNCE/12
  DemCounterPassedThreshold/1 -> AEMS_DEM_COUNTERBASEDDEBOUNCE/10
  DemCounterJumpUp/1 -> AEMS_DEM_COUNTERBASEDDEBOUNCE/8
  DemCounterJumpUpValue/1 -> AEMS_DEM_COUNTERBASEDDEBOUNCE/9
  DemCounterDecrementStepSize/1 -> AEMS_DEM_COUNTERBASEDDEBOUNCE/11
  DemCounterJumpDownValue/1 -> AEMS_DEM_COUNTERBASEDDEBOUNCE/13
  DemCounterIncrementStepSize/1 -> AEMS_DEM_COUNTERBASEDDEBOUNCE/7
  AEMS_DEM_COUNTERBASEDDEBOUNCE/3 -> passed/1
  AEMS_DEM_COUNTERBASEDDEBOUNCE/2 -> failed/1
  AEMS_DEM_COUNTERBASEDDEBOUNCE/1 -> debouncevalue/1
  prefailed/1 -> AEMS_DEM_COUNTERBASEDDEBOUNCE/2
  prepassed/1 -> AEMS_DEM_COUNTERBASEDDEBOUNCE/3
  conditionfulfilled/1 -> AEMS_DEM_COUNTERBASEDDEBOUNCE/1

== system AEMS_Standard_Library/SUB/AEMS_DEM_COUNTER_BASED_DEBOUNCE_8D/AEMS_DEM_COUNTER_BASED_DEBOUNCE_CALL2 ==
  conditionfulfilled : Inport
  prefailed : Inport  Port=2
  prepassed : Inport  Port=3
  reseteventdebounce : Inport  Port=4
  DemDebounceBehavior : Inport  Port=5
  DemCounterFailedThreshold : Inport  Port=6
  DemCounterIncrementStepSize : Inport  Port=7
  DemCounterJumpUp : Inport  Port=8
  DemCounterJumpUpValue : Inport  Port=9
  DemCounterPassedThreshold : Inport  Port=10
  DemCounterDecrementStepSize : Inport  Port=11
  DemCounterJumpDown : Inport  Port=12
  DemCounterJumpDownValue : Inport  Port=13
  Enable : EnablePort
  AEMS_DEM_COUNTERBASEDDEBOUNCE : AEMS_Standard_Library/SUB/AEMS_DEM_COUNTERBASEDDEBOUNCE  Tag=[LIB]  eventid=Dem_EventId_Device2_Faulttype
      settings: AttributesFormatString=|
      | %<MaskType>
      | EventId: %<eventid>
  debouncevalue : Outport
  failed : Outport  Port=2
  passed : Outport  Port=3
  wires:
  reseteventdebounce/1 -> AEMS_DEM_COUNTERBASEDDEBOUNCE/4
  DemCounterPassedThreshold/1 -> AEMS_DEM_COUNTERBASEDDEBOUNCE/10
  DemCounterDecrementStepSize/1 -> AEMS_DEM_COUNTERBASEDDEBOUNCE/11
  DemCounterJumpDown/1 -> AEMS_DEM_COUNTERBASEDDEBOUNCE/12
  DemCounterJumpUp/1 -> AEMS_DEM_COUNTERBASEDDEBOUNCE/8
  DemCounterFailedThreshold/1 -> AEMS_DEM_COUNTERBASEDDEBOUNCE/6
  DemDebounceBehavior/1 -> AEMS_DEM_COUNTERBASEDDEBOUNCE/5
  DemCounterIncrementStepSize/1 -> AEMS_DEM_COUNTERBASEDDEBOUNCE/7
  DemCounterJumpUpValue/1 -> AEMS_DEM_COUNTERBASEDDEBOUNCE/9
  DemCounterJumpDownValue/1 -> AEMS_DEM_COUNTERBASEDDEBOUNCE/13
  AEMS_DEM_COUNTERBASEDDEBOUNCE/3 -> passed/1
  AEMS_DEM_COUNTERBASEDDEBOUNCE/2 -> failed/1
  AEMS_DEM_COUNTERBASEDDEBOUNCE/1 -> debouncevalue/1
  prefailed/1 -> AEMS_DEM_COUNTERBASEDDEBOUNCE/2
  prepassed/1 -> AEMS_DEM_COUNTERBASEDDEBOUNCE/3
  conditionfulfilled/1 -> AEMS_DEM_COUNTERBASEDDEBOUNCE/1

== system AEMS_Standard_Library/SUB/AEMS_DEM_COUNTER_BASED_DEBOUNCE_8D/AEMS_DEM_COUNTER_BASED_DEBOUNCE_CALL3 ==
  conditionfulfilled : Inport
  prefailed : Inport  Port=2
  prepassed : Inport  Port=3
  reseteventdebounce : Inport  Port=4
  DemDebounceBehavior : Inport  Port=5
  DemCounterFailedThreshold : Inport  Port=6
  DemCounterIncrementStepSize : Inport  Port=7
  DemCounterJumpUp : Inport  Port=8
  DemCounterJumpUpValue : Inport  Port=9
  DemCounterPassedThreshold : Inport  Port=10
  DemCounterDecrementStepSize : Inport  Port=11
  DemCounterJumpDown : Inport  Port=12
  DemCounterJumpDownValue : Inport  Port=13
  Enable : EnablePort
  AEMS_DEM_COUNTERBASEDDEBOUNCE : AEMS_Standard_Library/SUB/AEMS_DEM_COUNTERBASEDDEBOUNCE  Tag=[LIB]  eventid=Dem_EventId_Device3_Faulttype
      settings: AttributesFormatString=|
      | %<MaskType>
      | EventId: %<eventid>
  debouncevalue : Outport
  failed : Outport  Port=2
  passed : Outport  Port=3
  wires:
  DemDebounceBehavior/1 -> AEMS_DEM_COUNTERBASEDDEBOUNCE/5
  DemCounterIncrementStepSize/1 -> AEMS_DEM_COUNTERBASEDDEBOUNCE/7
  DemCounterDecrementStepSize/1 -> AEMS_DEM_COUNTERBASEDDEBOUNCE/11
  DemCounterJumpDownValue/1 -> AEMS_DEM_COUNTERBASEDDEBOUNCE/13
  DemCounterJumpUpValue/1 -> AEMS_DEM_COUNTERBASEDDEBOUNCE/9
  DemCounterPassedThreshold/1 -> AEMS_DEM_COUNTERBASEDDEBOUNCE/10
  DemCounterJumpDown/1 -> AEMS_DEM_COUNTERBASEDDEBOUNCE/12
  DemCounterFailedThreshold/1 -> AEMS_DEM_COUNTERBASEDDEBOUNCE/6
  DemCounterJumpUp/1 -> AEMS_DEM_COUNTERBASEDDEBOUNCE/8
  reseteventdebounce/1 -> AEMS_DEM_COUNTERBASEDDEBOUNCE/4
  conditionfulfilled/1 -> AEMS_DEM_COUNTERBASEDDEBOUNCE/1
  prepassed/1 -> AEMS_DEM_COUNTERBASEDDEBOUNCE/3
  prefailed/1 -> AEMS_DEM_COUNTERBASEDDEBOUNCE/2
  AEMS_DEM_COUNTERBASEDDEBOUNCE/1 -> debouncevalue/1
  AEMS_DEM_COUNTERBASEDDEBOUNCE/2 -> failed/1
  AEMS_DEM_COUNTERBASEDDEBOUNCE/3 -> passed/1

== system AEMS_Standard_Library/SUB/AEMS_DEM_COUNTER_BASED_DEBOUNCE_8D/AEMS_DEM_COUNTER_BASED_DEBOUNCE_CALL4 ==
  conditionfulfilled : Inport
  prefailed : Inport  Port=2
  prepassed : Inport  Port=3
  reseteventdebounce : Inport  Port=4
  DemDebounceBehavior : Inport  Port=5
  DemCounterFailedThreshold : Inport  Port=6
  DemCounterIncrementStepSize : Inport  Port=7
  DemCounterJumpUp : Inport  Port=8
  DemCounterJumpUpValue : Inport  Port=9
  DemCounterPassedThreshold : Inport  Port=10
  DemCounterDecrementStepSize : Inport  Port=11
  DemCounterJumpDown : Inport  Port=12
  DemCounterJumpDownValue : Inport  Port=13
  Enable : EnablePort
  AEMS_DEM_COUNTERBASEDDEBOUNCE : AEMS_Standard_Library/SUB/AEMS_DEM_COUNTERBASEDDEBOUNCE  Tag=[LIB]  eventid=Dem_EventId_Device4_Faulttype
      settings: AttributesFormatString=|
      | %<MaskType>
      | EventId: %<eventid>
  debouncevalue : Outport
  failed : Outport  Port=2
  passed : Outport  Port=3
  wires:
  DemCounterPassedThreshold/1 -> AEMS_DEM_COUNTERBASEDDEBOUNCE/10
  DemCounterFailedThreshold/1 -> AEMS_DEM_COUNTERBASEDDEBOUNCE/6
  DemCounterIncrementStepSize/1 -> AEMS_DEM_COUNTERBASEDDEBOUNCE/7
  DemCounterJumpDown/1 -> AEMS_DEM_COUNTERBASEDDEBOUNCE/12
  DemCounterJumpUpValue/1 -> AEMS_DEM_COUNTERBASEDDEBOUNCE/9
  DemCounterJumpUp/1 -> AEMS_DEM_COUNTERBASEDDEBOUNCE/8
  DemCounterDecrementStepSize/1 -> AEMS_DEM_COUNTERBASEDDEBOUNCE/11
  reseteventdebounce/1 -> AEMS_DEM_COUNTERBASEDDEBOUNCE/4
  DemDebounceBehavior/1 -> AEMS_DEM_COUNTERBASEDDEBOUNCE/5
  DemCounterJumpDownValue/1 -> AEMS_DEM_COUNTERBASEDDEBOUNCE/13
  AEMS_DEM_COUNTERBASEDDEBOUNCE/3 -> passed/1
  AEMS_DEM_COUNTERBASEDDEBOUNCE/2 -> failed/1
  AEMS_DEM_COUNTERBASEDDEBOUNCE/1 -> debouncevalue/1
  prefailed/1 -> AEMS_DEM_COUNTERBASEDDEBOUNCE/2
  prepassed/1 -> AEMS_DEM_COUNTERBASEDDEBOUNCE/3
  conditionfulfilled/1 -> AEMS_DEM_COUNTERBASEDDEBOUNCE/1

== system AEMS_Standard_Library/SUB/AEMS_DEM_COUNTER_BASED_DEBOUNCE_8D/AEMS_DEM_COUNTER_BASED_DEBOUNCE_CALL5 ==
  conditionfulfilled : Inport
  prefailed : Inport  Port=2
  prepassed : Inport  Port=3
  reseteventdebounce : Inport  Port=4
  DemDebounceBehavior : Inport  Port=5
  DemCounterFailedThreshold : Inport  Port=6
  DemCounterIncrementStepSize : Inport  Port=7
  DemCounterJumpUp : Inport  Port=8
  DemCounterJumpUpValue : Inport  Port=9
  DemCounterPassedThreshold : Inport  Port=10
  DemCounterDecrementStepSize : Inport  Port=11
  DemCounterJumpDown : Inport  Port=12
  DemCounterJumpDownValue : Inport  Port=13
  Enable : EnablePort
  AEMS_DEM_COUNTERBASEDDEBOUNCE : AEMS_Standard_Library/SUB/AEMS_DEM_COUNTERBASEDDEBOUNCE  Tag=[LIB]  eventid=Dem_EventId_Device5_Faulttype
      settings: AttributesFormatString=|
      | %<MaskType>
      | EventId: %<eventid>
  debouncevalue : Outport
  failed : Outport  Port=2
  passed : Outport  Port=3
  wires:
  DemCounterIncrementStepSize/1 -> AEMS_DEM_COUNTERBASEDDEBOUNCE/7
  DemCounterJumpDown/1 -> AEMS_DEM_COUNTERBASEDDEBOUNCE/12
  DemCounterJumpUp/1 -> AEMS_DEM_COUNTERBASEDDEBOUNCE/8
  DemCounterPassedThreshold/1 -> AEMS_DEM_COUNTERBASEDDEBOUNCE/10
  DemCounterJumpDownValue/1 -> AEMS_DEM_COUNTERBASEDDEBOUNCE/13
  DemCounterDecrementStepSize/1 -> AEMS_DEM_COUNTERBASEDDEBOUNCE/11
  DemCounterJumpUpValue/1 -> AEMS_DEM_COUNTERBASEDDEBOUNCE/9
  DemCounterFailedThreshold/1 -> AEMS_DEM_COUNTERBASEDDEBOUNCE/6
  reseteventdebounce/1 -> AEMS_DEM_COUNTERBASEDDEBOUNCE/4
  DemDebounceBehavior/1 -> AEMS_DEM_COUNTERBASEDDEBOUNCE/5
  AEMS_DEM_COUNTERBASEDDEBOUNCE/3 -> passed/1
  AEMS_DEM_COUNTERBASEDDEBOUNCE/2 -> failed/1
  AEMS_DEM_COUNTERBASEDDEBOUNCE/1 -> debouncevalue/1
  prefailed/1 -> AEMS_DEM_COUNTERBASEDDEBOUNCE/2
  prepassed/1 -> AEMS_DEM_COUNTERBASEDDEBOUNCE/3
  conditionfulfilled/1 -> AEMS_DEM_COUNTERBASEDDEBOUNCE/1

== system AEMS_Standard_Library/SUB/AEMS_DEM_COUNTER_BASED_DEBOUNCE_8D/AEMS_DEM_COUNTER_BASED_DEBOUNCE_CALL6 ==
  conditionfulfilled : Inport
  prefailed : Inport  Port=2
  prepassed : Inport  Port=3
  reseteventdebounce : Inport  Port=4
  DemDebounceBehavior : Inport  Port=5
  DemCounterFailedThreshold : Inport  Port=6
  DemCounterIncrementStepSize : Inport  Port=7
  DemCounterJumpUp : Inport  Port=8
  DemCounterJumpUpValue : Inport  Port=9
  DemCounterPassedThreshold : Inport  Port=10
  DemCounterDecrementStepSize : Inport  Port=11
  DemCounterJumpDown : Inport  Port=12
  DemCounterJumpDownValue : Inport  Port=13
  Enable : EnablePort
  AEMS_DEM_COUNTERBASEDDEBOUNCE : AEMS_Standard_Library/SUB/AEMS_DEM_COUNTERBASEDDEBOUNCE  Tag=[LIB]  eventid=Dem_EventId_Device6_Faulttype
      settings: AttributesFormatString=|
      | %<MaskType>
      | EventId: %<eventid>
  debouncevalue : Outport
  failed : Outport  Port=2
  passed : Outport  Port=3
  wires:
  DemCounterDecrementStepSize/1 -> AEMS_DEM_COUNTERBASEDDEBOUNCE/11
  DemCounterJumpUp/1 -> AEMS_DEM_COUNTERBASEDDEBOUNCE/8
  reseteventdebounce/1 -> AEMS_DEM_COUNTERBASEDDEBOUNCE/4
  DemDebounceBehavior/1 -> AEMS_DEM_COUNTERBASEDDEBOUNCE/5
  DemCounterIncrementStepSize/1 -> AEMS_DEM_COUNTERBASEDDEBOUNCE/7
  DemCounterJumpUpValue/1 -> AEMS_DEM_COUNTERBASEDDEBOUNCE/9
  DemCounterJumpDownValue/1 -> AEMS_DEM_COUNTERBASEDDEBOUNCE/13
  DemCounterPassedThreshold/1 -> AEMS_DEM_COUNTERBASEDDEBOUNCE/10
  DemCounterJumpDown/1 -> AEMS_DEM_COUNTERBASEDDEBOUNCE/12
  DemCounterFailedThreshold/1 -> AEMS_DEM_COUNTERBASEDDEBOUNCE/6
  AEMS_DEM_COUNTERBASEDDEBOUNCE/3 -> passed/1
  AEMS_DEM_COUNTERBASEDDEBOUNCE/2 -> failed/1
  AEMS_DEM_COUNTERBASEDDEBOUNCE/1 -> debouncevalue/1
  prefailed/1 -> AEMS_DEM_COUNTERBASEDDEBOUNCE/2
  prepassed/1 -> AEMS_DEM_COUNTERBASEDDEBOUNCE/3
  conditionfulfilled/1 -> AEMS_DEM_COUNTERBASEDDEBOUNCE/1

== system AEMS_Standard_Library/SUB/AEMS_DEM_COUNTER_BASED_DEBOUNCE_8D/AEMS_DEM_COUNTER_BASED_DEBOUNCE_CALL7 ==
  conditionfulfilled : Inport
  prefailed : Inport  Port=2
  prepassed : Inport  Port=3
  reseteventdebounce : Inport  Port=4
  DemDebounceBehavior : Inport  Port=5
  DemCounterFailedThreshold : Inport  Port=6
  DemCounterIncrementStepSize : Inport  Port=7
  DemCounterJumpUp : Inport  Port=8
  DemCounterJumpUpValue : Inport  Port=9
  DemCounterPassedThreshold : Inport  Port=10
  DemCounterDecrementStepSize : Inport  Port=11
  DemCounterJumpDown : Inport  Port=12
  DemCounterJumpDownValue : Inport  Port=13
  Enable : EnablePort
  AEMS_DEM_COUNTERBASEDDEBOUNCE : AEMS_Standard_Library/SUB/AEMS_DEM_COUNTERBASEDDEBOUNCE  Tag=[LIB]  eventid=Dem_EventId_Device7_Faulttype
      settings: AttributesFormatString=|
      | %<MaskType>
      | EventId: %<eventid>
  debouncevalue : Outport
  failed : Outport  Port=2
  passed : Outport  Port=3
  wires:
  DemCounterIncrementStepSize/1 -> AEMS_DEM_COUNTERBASEDDEBOUNCE/7
  DemCounterJumpUpValue/1 -> AEMS_DEM_COUNTERBASEDDEBOUNCE/9
  DemCounterJumpUp/1 -> AEMS_DEM_COUNTERBASEDDEBOUNCE/8
  DemCounterFailedThreshold/1 -> AEMS_DEM_COUNTERBASEDDEBOUNCE/6
  DemCounterJumpDownValue/1 -> AEMS_DEM_COUNTERBASEDDEBOUNCE/13
  DemCounterDecrementStepSize/1 -> AEMS_DEM_COUNTERBASEDDEBOUNCE/11
  DemCounterPassedThreshold/1 -> AEMS_DEM_COUNTERBASEDDEBOUNCE/10
  DemCounterJumpDown/1 -> AEMS_DEM_COUNTERBASEDDEBOUNCE/12
  DemDebounceBehavior/1 -> AEMS_DEM_COUNTERBASEDDEBOUNCE/5
  reseteventdebounce/1 -> AEMS_DEM_COUNTERBASEDDEBOUNCE/4
  conditionfulfilled/1 -> AEMS_DEM_COUNTERBASEDDEBOUNCE/1
  prepassed/1 -> AEMS_DEM_COUNTERBASEDDEBOUNCE/3
  prefailed/1 -> AEMS_DEM_COUNTERBASEDDEBOUNCE/2
  AEMS_DEM_COUNTERBASEDDEBOUNCE/1 -> debouncevalue/1
  AEMS_DEM_COUNTERBASEDDEBOUNCE/2 -> failed/1
  AEMS_DEM_COUNTERBASEDDEBOUNCE/3 -> passed/1

== system AEMS_Standard_Library/SUB/AEMS_DEM_COUNTER_BASED_DEBOUNCE_8D/AEMS_DEM_COUNTER_BASED_DEBOUNCE_CALL8 ==
  conditionfulfilled : Inport
  prefailed : Inport  Port=2
  prepassed : Inport  Port=3
  reseteventdebounce : Inport  Port=4
  DemDebounceBehavior : Inport  Port=5
  DemCounterFailedThreshold : Inport  Port=6
  DemCounterIncrementStepSize : Inport  Port=7
  DemCounterJumpUp : Inport  Port=8
  DemCounterJumpUpValue : Inport  Port=9
  DemCounterPassedThreshold : Inport  Port=10
  DemCounterDecrementStepSize : Inport  Port=11
  DemCounterJumpDown : Inport  Port=12
  DemCounterJumpDownValue : Inport  Port=13
  Enable : EnablePort
  AEMS_DEM_COUNTERBASEDDEBOUNCE : AEMS_Standard_Library/SUB/AEMS_DEM_COUNTERBASEDDEBOUNCE  Tag=[LIB]  eventid=Dem_EventId_Device8_Faulttype
      settings: AttributesFormatString=|
      | %<MaskType>
      | EventId: %<eventid>
  debouncevalue : Outport
  failed : Outport  Port=2
  passed : Outport  Port=3
  wires:
  DemDebounceBehavior/1 -> AEMS_DEM_COUNTERBASEDDEBOUNCE/5
  DemCounterDecrementStepSize/1 -> AEMS_DEM_COUNTERBASEDDEBOUNCE/11
  DemCounterIncrementStepSize/1 -> AEMS_DEM_COUNTERBASEDDEBOUNCE/7
  DemCounterJumpUp/1 -> AEMS_DEM_COUNTERBASEDDEBOUNCE/8
  DemCounterJumpDownValue/1 -> AEMS_DEM_COUNTERBASEDDEBOUNCE/13
  DemCounterFailedThreshold/1 -> AEMS_DEM_COUNTERBASEDDEBOUNCE/6
  DemCounterPassedThreshold/1 -> AEMS_DEM_COUNTERBASEDDEBOUNCE/10
  DemCounterJumpUpValue/1 -> AEMS_DEM_COUNTERBASEDDEBOUNCE/9
  DemCounterJumpDown/1 -> AEMS_DEM_COUNTERBASEDDEBOUNCE/12
  reseteventdebounce/1 -> AEMS_DEM_COUNTERBASEDDEBOUNCE/4
  conditionfulfilled/1 -> AEMS_DEM_COUNTERBASEDDEBOUNCE/1
  prepassed/1 -> AEMS_DEM_COUNTERBASEDDEBOUNCE/3
  prefailed/1 -> AEMS_DEM_COUNTERBASEDDEBOUNCE/2
  AEMS_DEM_COUNTERBASEDDEBOUNCE/1 -> debouncevalue/1
  AEMS_DEM_COUNTERBASEDDEBOUNCE/2 -> failed/1
  AEMS_DEM_COUNTERBASEDDEBOUNCE/3 -> passed/1

== system AEMS_Standard_Library/SUB/AEMS_DEM_COUNTER_BASED_DEBOUNCE_THRSHOLD_DYN_1D/AEMS_DEM_COUNTER_BASED_DEBOUNCE_THRSHOLD_DYN_CALL ==
  conditionfulfilled : Inport
  prefailed : Inport  Port=2
  prepassed : Inport  Port=3
  DemDebounceBehavior : Inport  Port=4
  failedthreshold : Inport  Port=5
  DemCounterIncrementStepSize : Inport  Port=6
  DemCounterJumpUp : Inport  Port=7
  DemCounterJumpUpValue : Inport  Port=8
  passedthreshold : Inport  Port=9
  DemCounterDecrementStepSize : Inport  Port=10
  DemCounterJumpDown : Inport  Port=11
  DemCounterJumpDownValue : Inport  Port=12
  reseteventdebounce : Inport  Port=13
  Enable : EnablePort
      settings: AttributesFormatString=StatesWhenEnabling = %<StatesWhenEnabling>
  AEMS_DEM_COUNTERBASEDDEBOUNCE : AEMS_Standard_Library/SUB/AEMS_DEM_COUNTERBASEDDEBOUNCE  Tag=[LIB]  eventid=Dem_EventId_Device_Faulttype
      settings: AttributesFormatString=|
      | %<MaskType>
      | EventId: %<eventid>
  debouncevalue : Outport
      settings: AttributesFormatString=<initial=%<InitialOutput>>\n<whendisabled=%<OutputWhenDisabled>>
  failed : Outport  Port=2
      settings: AttributesFormatString=<initial=%<InitialOutput>>\n<whendisabled=%<OutputWhenDisabled>>
  passed : Outport  Port=3
      settings: AttributesFormatString=<initial=%<InitialOutput>>\n<whendisabled=%<OutputWhenDisabled>>
  wires:
  conditionfulfilled/1 -> AEMS_DEM_COUNTERBASEDDEBOUNCE/1
  prepassed/1 -> AEMS_DEM_COUNTERBASEDDEBOUNCE/3
  prefailed/1 -> AEMS_DEM_COUNTERBASEDDEBOUNCE/2
  AEMS_DEM_COUNTERBASEDDEBOUNCE/1 -> debouncevalue/1
  AEMS_DEM_COUNTERBASEDDEBOUNCE/2 -> failed/1
  AEMS_DEM_COUNTERBASEDDEBOUNCE/3 -> passed/1
  reseteventdebounce/1 -> AEMS_DEM_COUNTERBASEDDEBOUNCE/4
  DemCounterJumpDownValue/1 -> AEMS_DEM_COUNTERBASEDDEBOUNCE/13
  DemCounterJumpDown/1 -> AEMS_DEM_COUNTERBASEDDEBOUNCE/12
  DemCounterDecrementStepSize/1 -> AEMS_DEM_COUNTERBASEDDEBOUNCE/11
  passedthreshold/1 -> AEMS_DEM_COUNTERBASEDDEBOUNCE/10
  DemCounterJumpUpValue/1 -> AEMS_DEM_COUNTERBASEDDEBOUNCE/9
  DemCounterJumpUp/1 -> AEMS_DEM_COUNTERBASEDDEBOUNCE/8
  DemCounterIncrementStepSize/1 -> AEMS_DEM_COUNTERBASEDDEBOUNCE/7
  failedthreshold/1 -> AEMS_DEM_COUNTERBASEDDEBOUNCE/6
  DemDebounceBehavior/1 -> AEMS_DEM_COUNTERBASEDDEBOUNCE/5
